simulink model "EncoderTest"  (R2015a)
settings: Solver=ode3  StartTime=0.0  StopTime=10.0  RelTol=1e-3
libraries: PoliArd x6
settings Model: ExtModeTrigDuration=2  Creator=User  LastModifiedBy=User
settings OptimizationCC: OptimizeModelRefInitCode=on  LifeSpan=1
settings DebuggingCC: UnderspecifiedInitializationDetection=Classic  MergeDetectMultiDrivingBlocksExec=none
settings HardwareCC: ProdLargestAtomicInteger=Long  ProdLargestAtomicFloat=Double  ProdEndianess=LittleEndian  ProdHWDeviceType=ARM Compatible->ARM Cortex
settings RTWCC: SystemTargetFile=realtime.tlc  GenerateMakefile=off  TemplateMakefile=realtime.tmf  Description=Run on Target Hardware  RTWVerbose=off
settings ERTTargetCC: CombineOutputUpdateFcns=off  ExtModeTransport=3  ExtModeMexFile=ext_serial_win32_comm_rtt  ExtModeMexArgs=0 1 9600  ERTSrcFileBannerTemplate=realtime_code_template.cgt  ERTHdrFileBannerTemplate=realtime_code_template.cgt  ERTDataSrcFileTemplate=realtime_code_template.cgt  ERTDataHdrFileTemplate=realtime_code_template.cgt  ERTCustomFileTemplate=realtime_file_process.tlc

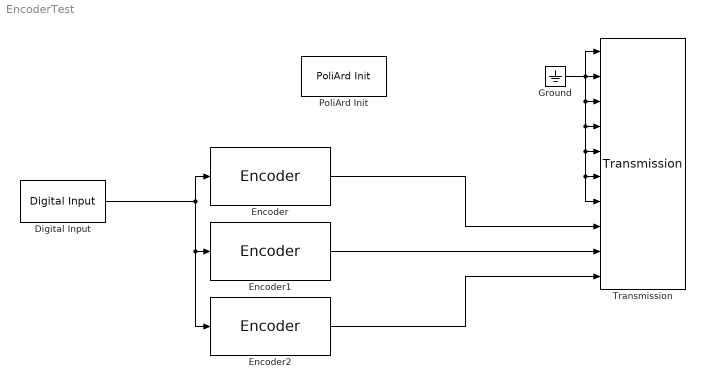
== system EncoderTest ==
  Digital Input : PoliArd/Digital Input  DI_pin=2  DIsample=-1
  Encoder : PoliArd/Encoder  EncoderID=1  dt_enc=-1
  Encoder1 : PoliArd/Encoder  EncoderID=4  dt_enc=-1
  Encoder2 : PoliArd/Encoder  EncoderID=3  dt_enc=-1
  Ground : Ground
  PoliArd Init : PoliArd/PoliArd Init
  Transmission : PoliArd/Transmission  sample_freq=100  sig_to_send=6
  wires:
  Digital Input/1 -> Encoder2/1, Encoder1/1, Encoder/1
  Encoder/1 -> Transmission/8
  Encoder1/1 -> Transmission/9
  Encoder2/1 -> Transmission/10
  Ground/1 -> Transmission/7, Transmission/6, Transmission/5, Transmission/4, Transmission/3, Transmission/1, Transmission/2
